simulink model "BasePerTracing"  (R2024b)
settings: Solver=FixedStepDiscrete  StartTime=0.0  StopTime=Inf  RelTol=1e-3  EnableMultiTasking=on
InitFcn:
  | mcb_pmsm_foc_qep_f28379d_data;
undefined symbols (not defined in the file): ADCCount, dataType, Down, GainVsense, GPTRIP1SEL, GPTRIP2SEL, J, Km, Kpi, Kpw, OffsetADCINC4, PulseNumber, RadiantsPerCount, RpmToRads, TaoFilterOffsetCurrent, TaoFilterOmega, Tii, Tiw, TSample, TZ1, TZ2, Up, VrefADC
libraries: c2802xlib x9, simulink x7, c280xlib x4, c2837xDlib x3, c2000lib x1, svdutilitieslib x1
(part 2 of 2)

== matlab function BasePerTracing/Current Control/ENCODER/MATLAB Function ==
  data: Ts input; out output; Tao input; In input
function out = LowPassFilter( Ts ,Tao, In)
persistent OutPrecedente
if isempty( OutPrecedente )
 OutPrecedente = 0 ;
end
% Filtro passa basso discretizzato con il
 % metodo delle differenze all'indietro

 a=Ts/(Ts+Tao);
 b=Tao/(Ts+Tao);

 out=a*In+OutPrecedente*b;

 OutPrecedente = out;

end

== matlab function BasePerTracing/Current Control/MATLAB Function1 ==
  settings: updateMethod=DISCRETE
  data: in input; out output; Kp input; Ti input; Ts input; Enable input; EnableCheckSat input; HiSat input; LowSat input; omega_m input
function out = PI( in ,Kp , Ti , Ts , Enable, EnableCheckSat, HiSat, LowSat, omega_m)
persistent in_prev out_prev
% Initial Value
if isempty( out_prev )
out_prev = 0;
end
if isempty( in_prev )
in_prev = 0;
end

% G(s)=(Kp/Ti)*((1+Ti*s)/s) (Tustin)
% We run control only if motor is running
if (Enable == 1)
%I Calculate the output
 out = Kp*Ts/(2*Ti)*(in+in_prev) + Kp*(in-in_prev) + out_prev ;
else
out = 0;
in = 0;
end

if(EnableCheckSat == 1)
%check for saturation
if out > HiSat
out = HiSat;
elseif (out < LowSat)
out = LowSat;
end
end

out_prev = out;
in_prev = in;
end

== matlab function BasePerTracing/Current Control/MATLAB Function2 ==
  settings: updateMethod=DISCRETE
  data: in input; out output; Kp input; Ti input; Ts input; Enable input; EnableCheckSat input; HiSat input; LowSat input; omega_m input
function out = PI( in ,Kp , Ti , Ts , Enable, EnableCheckSat, HiSat, LowSat, omega_m)
persistent in_prev out_prev
% Initial Value
if isempty( out_prev )
out_prev = 0;
end
if isempty( in_prev )
in_prev = 0;
end

% G(s)=(Kp/Ti)*((1+Ti*s)/s) (Tustin)
% We run control only if motor is running
if (Enable == 1)
%I Calculate the output
 out = Kp*Ts/(2*Ti)*(in+in_prev) + Kp*(in-in_prev) + out_prev ;
else
out = 0;
in = 0;
end

if(EnableCheckSat == 1)
%check for saturation
if out > HiSat
out = HiSat;
elseif (out < LowSat)
out = LowSat;
end
end

out_prev = out;
in_prev = in;
end
